simulink model "FuzzyModel"  (R2020a)
(part 3 of 4)

  "IW{1,1}(221,:)'"/1 -> dotprod221/1
  dotprod221/1 -> Mux/221
  "IW{1,1}(222,:)'"/1 -> dotprod222/1
  dotprod222/1 -> Mux/222
  "IW{1,1}(223,:)'"/1 -> dotprod223/1
  dotprod223/1 -> Mux/223
  "IW{1,1}(224,:)'"/1 -> dotprod224/1
  dotprod224/1 -> Mux/224
  "IW{1,1}(225,:)'"/1 -> dotprod225/1
  dotprod225/1 -> Mux/225
  "IW{1,1}(226,:)'"/1 -> dotprod226/1
  dotprod226/1 -> Mux/226
  "IW{1,1}(227,:)'"/1 -> dotprod227/1
  dotprod227/1 -> Mux/227
  "IW{1,1}(228,:)'"/1 -> dotprod228/1
  dotprod228/1 -> Mux/228
  "IW{1,1}(229,:)'"/1 -> dotprod229/1
  dotprod229/1 -> Mux/229
  "IW{1,1}(230,:)'"/1 -> dotprod230/1
  dotprod230/1 -> Mux/230
  "IW{1,1}(231,:)'"/1 -> dotprod231/1
  dotprod231/1 -> Mux/231
  "IW{1,1}(232,:)'"/1 -> dotprod232/1
  dotprod232/1 -> Mux/232
  "IW{1,1}(233,:)'"/1 -> dotprod233/1
  dotprod233/1 -> Mux/233
  "IW{1,1}(234,:)'"/1 -> dotprod234/1
  dotprod234/1 -> Mux/234
  "IW{1,1}(235,:)'"/1 -> dotprod235/1
  dotprod235/1 -> Mux/235
  "IW{1,1}(236,:)'"/1 -> dotprod236/1
  dotprod236/1 -> Mux/236
  "IW{1,1}(237,:)'"/1 -> dotprod237/1
  dotprod237/1 -> Mux/237
  "IW{1,1}(238,:)'"/1 -> dotprod238/1
  dotprod238/1 -> Mux/238
  "IW{1,1}(239,:)'"/1 -> dotprod239/1
  dotprod239/1 -> Mux/239
  "IW{1,1}(240,:)'"/1 -> dotprod240/1
  dotprod240/1 -> Mux/240
  "IW{1,1}(241,:)'"/1 -> dotprod241/1
  dotprod241/1 -> Mux/241
  "IW{1,1}(242,:)'"/1 -> dotprod242/1
  dotprod242/1 -> Mux/242
  "IW{1,1}(243,:)'"/1 -> dotprod243/1
  dotprod243/1 -> Mux/243
  "IW{1,1}(244,:)'"/1 -> dotprod244/1
  dotprod244/1 -> Mux/244
  "IW{1,1}(245,:)'"/1 -> dotprod245/1
  dotprod245/1 -> Mux/245
  "IW{1,1}(246,:)'"/1 -> dotprod246/1
  dotprod246/1 -> Mux/246
  "IW{1,1}(247,:)'"/1 -> dotprod247/1
  dotprod247/1 -> Mux/247
  "IW{1,1}(248,:)'"/1 -> dotprod248/1
  dotprod248/1 -> Mux/248
  "IW{1,1}(249,:)'"/1 -> dotprod249/1
  dotprod249/1 -> Mux/249
  "IW{1,1}(250,:)'"/1 -> dotprod250/1
  dotprod250/1 -> Mux/250
  Mux/1 -> "iz{1,1}"/1
